simulink model "thetaModify"  (R2019b)
settings: Solver=FixedStepAuto  StartTime=0.0  StopTime=10.0  FixedStep=0.1  RelTol=1e-3
settings Model: Creator=r720r  LastModifiedBy=r720r

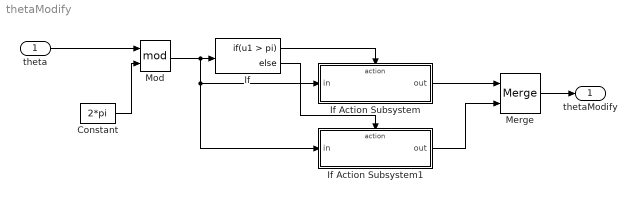
== system thetaModify ==
  theta : Inport  OutDataTypeStr=double  PortDimensions=1
  Constant : Constant  Value=2*pi
  If : If  IfExpression=u1 > pi
  If Action Subsystem : Subsystem  TreatAsAtomicUnit=on
  If Action Subsystem1 : Subsystem  TreatAsAtomicUnit=on
  Merge : Merge
  Mod : Math  Operator=mod  SignedPower=off  SaturateOnIntegerOverflow=on
  thetaModify : Outport
  wires:
  If Action Subsystem/1(out) -> Merge/1
  If/1 -> If Action Subsystem/Action
  If Action Subsystem1/1(out) -> Merge/2
  Mod/1 -> If Action Subsystem1/1(in), If Action Subsystem/1(in), If/1
  If/2 -> If Action Subsystem1/Action
  Constant/1 -> Mod/2
  Merge/1 -> thetaModify/1
  theta/1 -> Mod/1

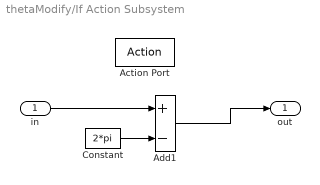
== system thetaModify/If Action Subsystem ==
  in : Inport
  Action Port : ActionPort  ActionPortLabel=if(u1 > pi)
  Add1 : Sum  Inputs=+-
  Constant : Constant  Value=2*pi
  out : Outport
  wires:
  in/1 -> Add1/1
  Add1/1 -> out/1
  Constant/1 -> Add1/2

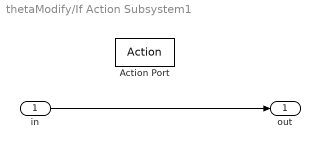
== system thetaModify/If Action Subsystem1 ==
  in : Inport
  Action Port : ActionPort  ActionPortLabel=else
  out : Outport
  wires:
  in/1 -> out/1
